simulink model "DC__motor"  (R2017a)
settings: Solver=ode3  StartTime=0.0  StopTime=5  FixedStep=.002  RelTol=1e-3  EnableMultiTasking=on
InitFcn:
  | Jm=0.01; % [kgm^2]
  | C=0.1;     % [Nms]
  | Ke=0.01;  % [Nm/A]
  | Kt=1;   % [Nm/A]
  | Ra=1.25;  % [Ohm]
  | La=0.5;     % [H]
settings Model: Creator=SLE  LastModifiedBy=sulaymon.eshkabilov
settings DataIOCC: SaveFormat=Array  SignalLoggingSaveFormat=ModelDataLogs
settings OptimizationCC: ExpressionDepthLimit=2147483647  LifeSpan=inf
settings DebuggingCC: UnderspecifiedInitializationDetection=Classic  MergeDetectMultiDrivingBlocksExec=none  SolverPrmCheckMsg=warning  FcnCallInpInsideContextMsg=warning  StateNameClashWarn=warning  SFUnexpectedBacktrackingDiag=warning  SFNoUnconditionalDefaultTransitionDiag=warning  SFExecutionAtInitializationDiag=none
settings HardwareCC: ProdBitPerPointer=32  ProdBitPerSizeT=32  ProdBitPerPtrDiffT=32  ProdLargestAtomicFloat=None  ProdIntDivRoundTo=Undefined  ProdEndianess=Unspecified  ProdWordSize=32  ProdHWDeviceType=32-bit Generic
settings ModelReferenceCC: PropagateSignalLabelsOutOfModel=off
settings RTWCC: GenCodeOnly=on  GenerateReport=on  TLCDebug=on  TLCAssert=on  RTWUseSimCustomCode=on  LaunchReport=on  TargetLang=C++
settings CodeAppCC: ForceParamTrailComments=on  UseSimReservedNames=on
settings GRTTargetCC: TargetLangStandard=C89/C90 (ANSI)  GeneratePreprocessorConditionals=Disable all  CombineOutputUpdateFcns=off  GRTInterface=on
settings ConfigComp: CovMetricSettings=dw  CovHtmlReporting=on  CovSaveCumulativeToWorkspaceVar=on  CovSaveSingleToWorkspaceVar=on  CovExternalEMLEnable=off

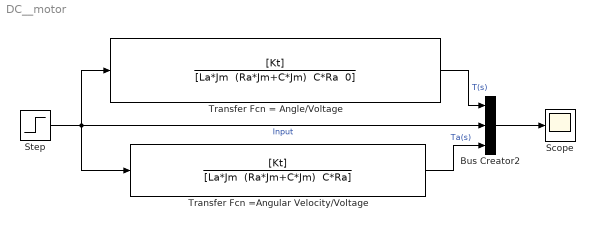
== system DC__motor ==
  Bus Creator2 : BusCreator  Inputs=3
  Scope : Scope
  Step : Step  After=12  SampleTime=0
  Transfer Fcn = Angle/Voltage : TransferFcn  Numerator=[Kt]  Denominator="[La*Jm  (Ra*Jm+C*Jm)  C*Ra  0]"
  Transfer Fcn =Angular Velocity/Voltage : TransferFcn  Numerator=[Kt]  Denominator="[La*Jm  (Ra*Jm+C*Jm)  C*Ra]"
  wires:
  Step/1 -> Bus Creator2/2, Transfer Fcn = Angle/Voltage/1, Transfer Fcn =Angular Velocity/Voltage/1  "Input"
  Bus Creator2/1 -> Scope/1
  Transfer Fcn = Angle/Voltage/1 -> Bus Creator2/1  "T(s)"
  Transfer Fcn =Angular Velocity/Voltage/1 -> Bus Creator2/3  "Ta(s)"
